simulink model "GUAM"  (R2023b)
settings: Solver=FixedStepAuto  StartTime=0.0  StopTime=SimIn.stopTime  FixedStep=Ts  RelTol=1e-3  AbsTol=1e-4  EnableMultiTasking=on
PostLoadFcn:
  | warning('off','sm:sli:setup:compile:LocalSolverNotSupported')
StartFcn:
  | tic
StopFcn:
  | Elapsed_Sim_Time = toc;
model workspace: external: MATLAB File aileronAssembly_DataFile.m (data not in the file)
values from neighbouring files (symbols this model uses):
  Ts = 0.05    [RUNME.m]
undefined symbols (not defined in the file or in its folder): AAC_Param, ang2Ext_coeff, Ki, Ki_scaling_elec, Kp, Leadscrew, motor_friction, R7_sctrl, sigbuilder_block, SimIn, SimPar, sm_aileron_actuator_lib, smiData, X, Y, Z
libraries: sm_lib x608, fl_lib x378, ee_lib x105, nesl_utility x96, simulink x10, eeGeneralControl x7, sh_lib x7, dspstat3 x6, sdl_lib x3, slpidlib x2, aerolibfltsims x2
(part 9 of 22)

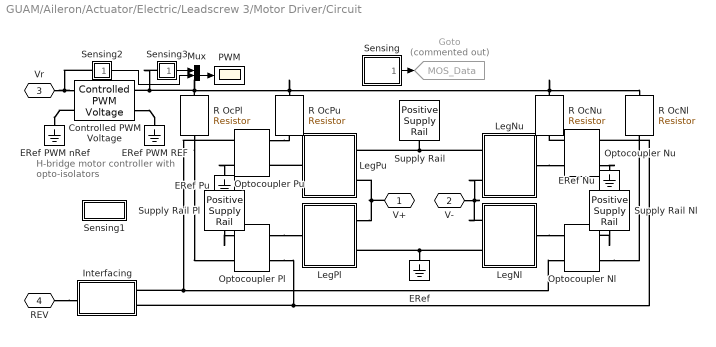
== system GUAM/Aileron/Actuator/Electric/Leadscrew 3/Motor Driver/Circuit ==
  note: H-bridge motor controller
      | with opto-isolators
  Controlled PWM Voltage : ee_lib/Integrated Circuits/Controlled PWM Voltage  F=10000 Hz  TD=0 s  pulse_width_offset=0 s  pulse_min=0 s  pwm_or_av=2  event_type=1  sample_time=1e-6 s  Vmin=0 V  Vmax=5 V  Vm=5 V  u_min=0  u_max=1
  ERef : fl_lib/Electrical/Electrical Elements/Electrical Reference
  ERef PWM REF : fl_lib/Electrical/Electrical Elements/Electrical Reference
  ERef PWM nRef : fl_lib/Electrical/Electrical Elements/Electrical Reference
  ERef Nu : fl_lib/Electrical/Electrical Elements/Electrical Reference
  ERef Pu : fl_lib/Electrical/Electrical Elements/Electrical Reference
  Goto : Goto  Commented=on  GotoTag=MOS_Data  TagVisibility=global
  Interfacing : Subsystem
  LegNl : Subsystem
      mask Display:
      | patch([96+30;0-30;0-30;96+30], [0+10;0+10;227-10;227-10], [1;1;1])
      | plot([96.6109160799533;96.4198282107139;95.8484048836359;94.9021492177306;93.5901741723367;91.9251147843401;89.9230064858609;87.6031306742773;84.9878290218281;82.1022883130956;78.9742978825019;75.6339819878271;72.1135096971394;68.4467850830839;64.6691207081296;60.8168975452888;56.927214609459;53.0375316736292;49.1853085107884;45.4076441358342;41.7409195217787;38.220447231091;34.8801313364162;31.7521409058224;28.86660019709;26.2512985446407;23.9314227330572;21.929314434578;20.2642550465813;18.9522800011875;18.0060243352822;17.4346010082041;17.2435131389648;17.4346010082041;18.0060243352822;18.9522800011875;20.2642550465814;21.9293144345781;23.9314227330573;26.2512985446408;28.8666001970901;31.7521409058226;34.8801313364163;38.2204472310911;41.7409195217788;45.4076441358342;49.1853085107884;53.0375316736292;56.927214609459;60.8168975452889;64.6691207081297;68.4467850830839;72.1135096971393;75.633981987827;78.9742978825018;82.1022883130955;84.9878290218281;87.6031306742773;89.9230064858608;91.9251147843399;93.5901741723367;94.9021492177305;95.8484048836358;96.4198282107139;96.6109160799533;96.6109160799533], [113.618216710165;109.728533774335;105.876310611494;102.09864623654;98.4319216224848;94.9114493317971;91.5711334371223;88.4431430065286;85.5576022977961;82.9423006453468;80.6224248337633;78.6203165352841;76.9552571472875;75.6432821018936;74.6970264359883;74.1256031089102;73.9345152396709;74.1256031089102;74.6970264359883;75.6432821018936;76.9552571472875;78.6203165352842;80.6224248337634;82.9423006453469;85.5576022977961;88.4431430065287;91.5711334371223;94.9114493317971;98.4319216224849;102.09864623654;105.876310611495;109.728533774335;113.618216710165;117.507899645995;121.360122808836;125.13778718379;128.804511797846;132.324984088533;135.665299983208;138.793290413802;141.678831122534;144.294132774983;146.614008586567;148.616116885046;150.281176273043;151.593151318437;152.539406984342;153.11083031142;153.301918180659;153.11083031142;152.539406984342;151.593151318437;150.281176273043;148.616116885046;146.614008586567;144.294132774983;141.678831122534;138.793290413802;135.665299983208;132.324984088533;128.804511797846;125.13778718379;121.360122808836;117.507899645995;113.618216710165;113.618216710165])
      | plot([33.9988537598401;34.5027737785131], [113.618216710165;113.618216710165])
      | plot([0.236212508752942;34.2508137691766], [113.618216710165;113.618216710165])
      | plot([34.2508137691766;34.2508137691766], [136.294617550448;90.9418158698827])
      | plot([45.5890141893178;45.5890141893178], [136.294617550448;90.9418158698827])
      | plot([45.5890141893178;68.2654150296003], [130.625517340377;130.625517340377])
      | plot([68.2654150296003;68.2654150296003], [130.625517340377;170.309218810871])
      | plot([68.2654150296003;93.776365974918], [170.309218810871;170.309218810871])
      | plot([45.5890141893178;68.2654150296003], [96.6109160799533;96.6109160799533])
      | plot([68.2654150296003;68.2654150296003], [96.6109160799533;56.927214609459])
      | plot([68.2654150296003;96.6109160799533], [56.927214609459;56.927214609459])
      | plot([45.5890141893178;68.2654150296003], [113.618216710165;113.618216710165])
      | plot([68.2654150296003;68.2654150296003], [130.618216710165;113.6109160799533])
      | plot([51.5963148195297;62.2581143993884;51.5963148195297], [124.956417130306;113.618216710165;102.280016290024])
  LegNu : Subsystem
      mask Display:
      | patch([96+30;0-30;0-30;96+30], [0+10;0+10;227-10;227-10], [1;1;1])
      | plot([96.6109160799533;96.4198282107139;95.8484048836359;94.9021492177306;93.5901741723367;91.9251147843401;89.9230064858609;87.6031306742773;84.9878290218281;82.1022883130956;78.9742978825019;75.6339819878271;72.1135096971394;68.4467850830839;64.6691207081296;60.8168975452888;56.927214609459;53.0375316736292;49.1853085107884;45.4076441358342;41.7409195217787;38.220447231091;34.8801313364162;31.7521409058224;28.86660019709;26.2512985446407;23.9314227330572;21.929314434578;20.2642550465813;18.9522800011875;18.0060243352822;17.4346010082041;17.2435131389648;17.4346010082041;18.0060243352822;18.9522800011875;20.2642550465814;21.9293144345781;23.9314227330573;26.2512985446408;28.8666001970901;31.7521409058226;34.8801313364163;38.2204472310911;41.7409195217788;45.4076441358342;49.1853085107884;53.0375316736292;56.927214609459;60.8168975452889;64.6691207081297;68.4467850830839;72.1135096971393;75.633981987827;78.9742978825018;82.1022883130955;84.9878290218281;87.6031306742773;89.9230064858608;91.9251147843399;93.5901741723367;94.9021492177305;95.8484048836358;96.4198282107139;96.6109160799533;96.6109160799533], [113.618216710165;109.728533774335;105.876310611494;102.09864623654;98.4319216224848;94.9114493317971;91.5711334371223;88.4431430065286;85.5576022977961;82.9423006453468;80.6224248337633;78.6203165352841;76.9552571472875;75.6432821018936;74.6970264359883;74.1256031089102;73.9345152396709;74.1256031089102;74.6970264359883;75.6432821018936;76.9552571472875;78.6203165352842;80.6224248337634;82.9423006453469;85.5576022977961;88.4431430065287;91.5711334371223;94.9114493317971;98.4319216224849;102.09864623654;105.876310611495;109.728533774335;113.618216710165;117.507899645995;121.360122808836;125.13778718379;128.804511797846;132.324984088533;135.665299983208;138.793290413802;141.678831122534;144.294132774983;146.614008586567;148.616116885046;150.281176273043;151.593151318437;152.539406984342;153.11083031142;153.301918180659;153.11083031142;152.539406984342;151.593151318437;150.281176273043;148.616116885046;146.614008586567;144.294132774983;141.678831122534;138.793290413802;135.665299983208;132.324984088533;128.804511797846;125.13778718379;121.360122808836;117.507899645995;113.618216710165;113.618216710165])
      | plot([33.9988537598401;34.5027737785131], [113.618216710165;113.618216710165])
      | plot([0.236212508752942;34.2508137691766], [113.618216710165;113.618216710165])
      | plot([34.2508137691766;34.2508137691766], [136.294617550448;90.9418158698827])
      | plot([45.5890141893178;45.5890141893178], [136.294617550448;90.9418158698827])
      | plot([45.5890141893178;68.2654150296003], [130.625517340377;130.625517340377])
      | plot([68.2654150296003;68.2654150296003], [130.625517340377;170.309218810871])
      | plot([68.2654150296003;93.776365974918], [170.309218810871;170.309218810871])
      | plot([45.5890141893178;68.2654150296003], [96.6109160799533;96.6109160799533])
      | plot([68.2654150296003;68.2654150296003], [96.6109160799533;56.927214609459])
      | plot([68.2654150296003;96.6109160799533], [56.927214609459;56.927214609459])
      | plot([45.5890141893178;68.2654150296003], [113.618216710165;113.618216710165])
      | plot([68.2654150296003;68.2654150296003], [130.618216710165;113.6109160799533])
      | plot([51.5963148195297;62.2581143993884;51.5963148195297], [124.956417130306;113.618216710165;102.280016290024])
  LegPl : Subsystem
      mask Display:
      | patch([96+30;0-30;0-30;96+30], [0+10;0+10;227-10;227-10], [1;1;1])
      | plot([96.6109160799533;96.4198282107139;95.8484048836359;94.9021492177306;93.5901741723367;91.9251147843401;89.9230064858609;87.6031306742773;84.9878290218281;82.1022883130956;78.9742978825019;75.6339819878271;72.1135096971394;68.4467850830839;64.6691207081296;60.8168975452888;56.927214609459;53.0375316736292;49.1853085107884;45.4076441358342;41.7409195217787;38.220447231091;34.8801313364162;31.7521409058224;28.86660019709;26.2512985446407;23.9314227330572;21.929314434578;20.2642550465813;18.9522800011875;18.0060243352822;17.4346010082041;17.2435131389648;17.4346010082041;18.0060243352822;18.9522800011875;20.2642550465814;21.9293144345781;23.9314227330573;26.2512985446408;28.8666001970901;31.7521409058226;34.8801313364163;38.2204472310911;41.7409195217788;45.4076441358342;49.1853085107884;53.0375316736292;56.927214609459;60.8168975452889;64.6691207081297;68.4467850830839;72.1135096971393;75.633981987827;78.9742978825018;82.1022883130955;84.9878290218281;87.6031306742773;89.9230064858608;91.9251147843399;93.5901741723367;94.9021492177305;95.8484048836358;96.4198282107139;96.6109160799533;96.6109160799533], [113.618216710165;109.728533774335;105.876310611494;102.09864623654;98.4319216224848;94.9114493317971;91.5711334371223;88.4431430065286;85.5576022977961;82.9423006453468;80.6224248337633;78.6203165352841;76.9552571472875;75.6432821018936;74.6970264359883;74.1256031089102;73.9345152396709;74.1256031089102;74.6970264359883;75.6432821018936;76.9552571472875;78.6203165352842;80.6224248337634;82.9423006453469;85.5576022977961;88.4431430065287;91.5711334371223;94.9114493317971;98.4319216224849;102.09864623654;105.876310611495;109.728533774335;113.618216710165;117.507899645995;121.360122808836;125.13778718379;128.804511797846;132.324984088533;135.665299983208;138.793290413802;141.678831122534;144.294132774983;146.614008586567;148.616116885046;150.281176273043;151.593151318437;152.539406984342;153.11083031142;153.301918180659;153.11083031142;152.539406984342;151.593151318437;150.281176273043;148.616116885046;146.614008586567;144.294132774983;141.678831122534;138.793290413802;135.665299983208;132.324984088533;128.804511797846;125.13778718379;121.360122808836;117.507899645995;113.618216710165;113.618216710165])
      | plot([33.9988537598401;34.5027737785131], [113.618216710165;113.618216710165])
      | plot([0.236212508752942;34.2508137691766], [113.618216710165;113.618216710165])
      | plot([34.2508137691766;34.2508137691766], [136.294617550448;90.9418158698827])
      | plot([45.5890141893178;45.5890141893178], [136.294617550448;90.9418158698827])
      | plot([45.5890141893178;68.2654150296003], [130.625517340377;130.625517340377])
      | plot([68.2654150296003;68.2654150296003], [130.625517340377;170.309218810871])
      | plot([68.2654150296003;93.776365974918], [170.309218810871;170.309218810871])
      | plot([45.5890141893178;68.2654150296003], [96.6109160799533;96.6109160799533])
      | plot([68.2654150296003;68.2654150296003], [96.6109160799533;56.927214609459])
      | plot([68.2654150296003;96.6109160799533], [56.927214609459;56.927214609459])
      | plot([45.5890141893178;68.2654150296003], [113.618216710165;113.618216710165])
      | plot([68.2654150296003;68.2654150296003], [130.618216710165;113.6109160799533])
      | plot([51.5963148195297;62.2581143993884;51.5963148195297], [124.956417130306;113.618216710165;102.280016290024])
  LegPu : Subsystem
      mask Display:
      | patch([96+30;0-30;0-30;96+30], [0+10;0+10;227-10;227-10], [1;1;1])
      | plot([96.6109160799533;96.4198282107139;95.8484048836359;94.9021492177306;93.5901741723367;91.9251147843401;89.9230064858609;87.6031306742773;84.9878290218281;82.1022883130956;78.9742978825019;75.6339819878271;72.1135096971394;68.4467850830839;64.6691207081296;60.8168975452888;56.927214609459;53.0375316736292;49.1853085107884;45.4076441358342;41.7409195217787;38.220447231091;34.8801313364162;31.7521409058224;28.86660019709;26.2512985446407;23.9314227330572;21.929314434578;20.2642550465813;18.9522800011875;18.0060243352822;17.4346010082041;17.2435131389648;17.4346010082041;18.0060243352822;18.9522800011875;20.2642550465814;21.9293144345781;23.9314227330573;26.2512985446408;28.8666001970901;31.7521409058226;34.8801313364163;38.2204472310911;41.7409195217788;45.4076441358342;49.1853085107884;53.0375316736292;56.927214609459;60.8168975452889;64.6691207081297;68.4467850830839;72.1135096971393;75.633981987827;78.9742978825018;82.1022883130955;84.9878290218281;87.6031306742773;89.9230064858608;91.9251147843399;93.5901741723367;94.9021492177305;95.8484048836358;96.4198282107139;96.6109160799533;96.6109160799533], [113.618216710165;109.728533774335;105.876310611494;102.09864623654;98.4319216224848;94.9114493317971;91.5711334371223;88.4431430065286;85.5576022977961;82.9423006453468;80.6224248337633;78.6203165352841;76.9552571472875;75.6432821018936;74.6970264359883;74.1256031089102;73.9345152396709;74.1256031089102;74.6970264359883;75.6432821018936;76.9552571472875;78.6203165352842;80.6224248337634;82.9423006453469;85.5576022977961;88.4431430065287;91.5711334371223;94.9114493317971;98.4319216224849;102.09864623654;105.876310611495;109.728533774335;113.618216710165;117.507899645995;121.360122808836;125.13778718379;128.804511797846;132.324984088533;135.665299983208;138.793290413802;141.678831122534;144.294132774983;146.614008586567;148.616116885046;150.281176273043;151.593151318437;152.539406984342;153.11083031142;153.301918180659;153.11083031142;152.539406984342;151.593151318437;150.281176273043;148.616116885046;146.614008586567;144.294132774983;141.678831122534;138.793290413802;135.665299983208;132.324984088533;128.804511797846;125.13778718379;121.360122808836;117.507899645995;113.618216710165;113.618216710165])
      | plot([33.9988537598401;34.5027737785131], [113.618216710165;113.618216710165])
      | plot([0.236212508752942;34.2508137691766], [113.618216710165;113.618216710165])
      | plot([34.2508137691766;34.2508137691766], [136.294617550448;90.9418158698827])
      | plot([45.5890141893178;45.5890141893178], [136.294617550448;90.9418158698827])
      | plot([45.5890141893178;68.2654150296003], [130.625517340377;130.625517340377])
      | plot([68.2654150296003;68.2654150296003], [130.625517340377;170.309218810871])
      | plot([68.2654150296003;93.776365974918], [170.309218810871;170.309218810871])
      | plot([45.5890141893178;68.2654150296003], [96.6109160799533;96.6109160799533])
      | plot([68.2654150296003;68.2654150296003], [96.6109160799533;56.927214609459])
      | plot([68.2654150296003;96.6109160799533], [56.927214609459;56.927214609459])
      | plot([45.5890141893178;68.2654150296003], [113.618216710165;113.618216710165])
      | plot([68.2654150296003;68.2654150296003], [130.618216710165;113.6109160799533])
      | plot([51.5963148195297;62.2581143993884;51.5963148195297], [124.956417130306;113.618216710165;102.280016290024])
  Mux : Mux  Inputs=2
  Optocoupler Nl : ee_lib/Semiconductors & Converters/Optocoupler  CTR=0.2  prmExp=1  I12="[  0.001 0.015 ] A"  V12="[  0.9 1.05 ] V"  IS=1e-10 A  ec=2  RS=0 Ohm  Tmeas=298.15 K  C_param=1  CJ=50 pF  CJ0=50 pF  VJ=1 V  Mgrad=0.5  Vvec="[  0.1 10 100 ] V"  Cvec="[  3.5 1 0.4 ] pF"  FC=0.5  T_param=1  IS_T2=1.8e-8 A  I1_T2=0.029 A  V1_T2=1.05 V  Tmeas2=125 degC  EG_param=1  EG=1.11 eV  XTI_param=1  XTI=3  Tdevice=25 degC  i_specify=off  i_priority=None  i=0 A  i_nominal_specify=off  i_nominal_unit=A  i_nominal_value=1  v_specify=off  v_priority=None  v=0 V  v_nominal_specify=off  v_nominal_unit=V  v_nominal_value=1  v_capacitor_specify=off  v_capacitor_priority=None  v_capacitor=0 V  v_capacitor_nominal_specify=off  v_capacitor_nominal_unit=V  v_capacitor_nominal_value=1  thermal_network_parameterization=ee.enum.thermalNetworkTopology.junctionCase  Rth=[0, 10] K/W  Rth_Cauer=[1, 3, 10] K/W  Rth_Foster=[4, 6] K/W  thermal_mass_parameterization=ee.enum.thermalNetwork.timeconstant  thermal_mass=[0, 1] J/K  thermal_mass_Cauer=[.1, .3, 1] J/K  thermal_mass_Foster=[1.5, 3] J/K  thermal_time_constant=[0, 10] s  thermal_time_constant_Cauer=[1, 3, 10] s  thermal_time_constant_Foster=[6, 18] s  thermal_mass_initial_temperatures=[25, 25] degC  thermal_mass_initial_temperatures_Cauer=[25, 25, 25] degC  Tvec_initial_Foster=[25, 25, 25, 25] degC  i_capacitor_specify=off  i_capacitor_priority=High  i_capacitor=0 A  i_capacitor_nominal_specify=off  i_capacitor_nominal_unit=A  i_capacitor_nominal_value=1
      settings: InternalSimscapePortConfiguration="{\"Bottom\":[],\"Left\":[{\"id\":\"p\",\"label\":\"\",\"type\":\"foundation.electrical.electrical\"},{\"id\":\"C\",\"label\":\"\",\"type\":\"foundation.electrical.electrical\"}],\"Right\":[{\"id\":\"n\",\"label\":\"\",\"type\":\"foundation.electrical.electrical\"},{\"id\":\"E\",\"label\":\"\",\"type\":\"foundation.electrical.electrical\"}],\"Top\":[]}"
  Optocoupler Nu : ee_lib/Semiconductors & Converters/Optocoupler  CTR=0.2  prmExp=1  I12="[  0.001 0.015 ] A"  V12="[  0.9 1.05 ] V"  IS=1e-10 A  ec=2  RS=0 Ohm  Tmeas=298.15 K  C_param=1  CJ=50 pF  CJ0=50 pF  VJ=1 V  Mgrad=0.5  Vvec="[  0.1 10 100 ] V"  Cvec="[  3.5 1 0.4 ] pF"  FC=0.5  T_param=1  IS_T2=1.8e-8 A  I1_T2=0.029 A  V1_T2=1.05 V  Tmeas2=125 degC  EG_param=1  EG=1.11 eV  XTI_param=1  XTI=3  Tdevice=25 degC  i_specify=off  i_priority=None  i=0 A  i_nominal_specify=off  i_nominal_unit=A  i_nominal_value=1  v_specify=off  v_priority=None  v=0 V  v_nominal_specify=off  v_nominal_unit=V  v_nominal_value=1  v_capacitor_specify=off  v_capacitor_priority=None  v_capacitor=0 V  v_capacitor_nominal_specify=off  v_capacitor_nominal_unit=V  v_capacitor_nominal_value=1  thermal_network_parameterization=ee.enum.thermalNetworkTopology.junctionCase  Rth=[0, 10] K/W  Rth_Cauer=[1, 3, 10] K/W  Rth_Foster=[4, 6] K/W  thermal_mass_parameterization=ee.enum.thermalNetwork.timeconstant  thermal_mass=[0, 1] J/K  thermal_mass_Cauer=[.1, .3, 1] J/K  thermal_mass_Foster=[1.5, 3] J/K  thermal_time_constant=[0, 10] s  thermal_time_constant_Cauer=[1, 3, 10] s  thermal_time_constant_Foster=[6, 18] s  thermal_mass_initial_temperatures=[25, 25] degC  thermal_mass_initial_temperatures_Cauer=[25, 25, 25] degC  Tvec_initial_Foster=[25, 25, 25, 25] degC  i_capacitor_specify=off  i_capacitor_priority=High  i_capacitor=0 A  i_capacitor_nominal_specify=off  i_capacitor_nominal_unit=A  i_capacitor_nominal_value=1
      settings: InternalSimscapePortConfiguration="{\"Bottom\":[],\"Left\":[{\"id\":\"p\",\"label\":\"\",\"type\":\"foundation.electrical.electrical\"},{\"id\":\"C\",\"label\":\"\",\"type\":\"foundation.electrical.electrical\"}],\"Right\":[{\"id\":\"n\",\"label\":\"\",\"type\":\"foundation.electrical.electrical\"},{\"id\":\"E\",\"label\":\"\",\"type\":\"foundation.electrical.electrical\"}],\"Top\":[]}"
  Optocoupler Pl : ee_lib/Semiconductors & Converters/Optocoupler  CTR=0.2  prmExp=1  I12="[  0.001 0.015 ] A"  V12="[  0.9 1.05 ] V"  IS=1e-10 A  ec=2  RS=0 Ohm  Tmeas=298.15 K  C_param=1  CJ=50 pF  CJ0=50 pF  VJ=1 V  Mgrad=0.5  Vvec="[  0.1 10 100 ] V"  Cvec="[  3.5 1 0.4 ] pF"  FC=0.5  T_param=1  IS_T2=1.8e-8 A  I1_T2=0.029 A  V1_T2=1.05 V  Tmeas2=125 degC  EG_param=1  EG=1.11 eV  XTI_param=1  XTI=3  Tdevice=25 degC  i_specify=off  i_priority=None  i=0 A  i_nominal_specify=off  i_nominal_unit=A  i_nominal_value=1  v_specify=off  v_priority=None  v=0 V  v_nominal_specify=off  v_nominal_unit=V  v_nominal_value=1  v_capacitor_specify=off  v_capacitor_priority=None  v_capacitor=0 V  v_capacitor_nominal_specify=off  v_capacitor_nominal_unit=V  v_capacitor_nominal_value=1  thermal_network_parameterization=ee.enum.thermalNetworkTopology.junctionCase  Rth=[0, 10] K/W  Rth_Cauer=[1, 3, 10] K/W  Rth_Foster=[4, 6] K/W  thermal_mass_parameterization=ee.enum.thermalNetwork.timeconstant  thermal_mass=[0, 1] J/K  thermal_mass_Cauer=[.1, .3, 1] J/K  thermal_mass_Foster=[1.5, 3] J/K  thermal_time_constant=[0, 10] s  thermal_time_constant_Cauer=[1, 3, 10] s  thermal_time_constant_Foster=[6, 18] s  thermal_mass_initial_temperatures=[25, 25] degC  thermal_mass_initial_temperatures_Cauer=[25, 25, 25] degC  Tvec_initial_Foster=[25, 25, 25, 25] degC  i_capacitor_specify=off  i_capacitor_priority=High  i_capacitor=0 A  i_capacitor_nominal_specify=off  i_capacitor_nominal_unit=A  i_capacitor_nominal_value=1
      settings: InternalSimscapePortConfiguration="{\"Bottom\":[],\"Left\":[{\"id\":\"p\",\"label\":\"\",\"type\":\"foundation.electrical.electrical\"},{\"id\":\"C\",\"label\":\"\",\"type\":\"foundation.electrical.electrical\"}],\"Right\":[{\"id\":\"n\",\"label\":\"\",\"type\":\"foundation.electrical.electrical\"},{\"id\":\"E\",\"label\":\"\",\"type\":\"foundation.electrical.electrical\"}],\"Top\":[]}"
  Optocoupler Pu : ee_lib/Semiconductors & Converters/Optocoupler  CTR=0.2  prmExp=1  I12="[  0.001 0.015 ] A"  V12="[  0.9 1.05 ] V"  IS=1e-10 A  ec=2  RS=0 Ohm  Tmeas=298.15 K  C_param=1  CJ=50 pF  CJ0=50 pF  VJ=1 V  Mgrad=0.5  Vvec="[  0.1 10 100 ] V"  Cvec="[  3.5 1 0.4 ] pF"  FC=0.5  T_param=1  IS_T2=1.8e-8 A  I1_T2=0.029 A  V1_T2=1.05 V  Tmeas2=125 degC  EG_param=1  EG=1.11 eV  XTI_param=1  XTI=3  Tdevice=25 degC  i_specify=off  i_priority=None  i=0 A  i_nominal_specify=off  i_nominal_unit=A  i_nominal_value=1  v_specify=off  v_priority=None  v=0 V  v_nominal_specify=off  v_nominal_unit=V  v_nominal_value=1  v_capacitor_specify=off  v_capacitor_priority=None  v_capacitor=0 V  v_capacitor_nominal_specify=off  v_capacitor_nominal_unit=V  v_capacitor_nominal_value=1  thermal_network_parameterization=ee.enum.thermalNetworkTopology.junctionCase  Rth=[0, 10] K/W  Rth_Cauer=[1, 3, 10] K/W  Rth_Foster=[4, 6] K/W  thermal_mass_parameterization=ee.enum.thermalNetwork.timeconstant  thermal_mass=[0, 1] J/K  thermal_mass_Cauer=[.1, .3, 1] J/K  thermal_mass_Foster=[1.5, 3] J/K  thermal_time_constant=[0, 10] s  thermal_time_constant_Cauer=[1, 3, 10] s  thermal_time_constant_Foster=[6, 18] s  thermal_mass_initial_temperatures=[25, 25] degC  thermal_mass_initial_temperatures_Cauer=[25, 25, 25] degC  Tvec_initial_Foster=[25, 25, 25, 25] degC  i_capacitor_specify=off  i_capacitor_priority=High  i_capacitor=0 A  i_capacitor_nominal_specify=off  i_capacitor_nominal_unit=A  i_capacitor_nominal_value=1
      settings: InternalSimscapePortConfiguration="{\"Bottom\":[],\"Left\":[{\"id\":\"p\",\"label\":\"\",\"type\":\"foundation.electrical.electrical\"},{\"id\":\"C\",\"label\":\"\",\"type\":\"foundation.electrical.electrical\"}],\"Right\":[{\"id\":\"n\",\"label\":\"\",\"type\":\"foundation.electrical.electrical\"},{\"id\":\"E\",\"label\":\"\",\"type\":\"foundation.electrical.electrical\"}],\"Top\":[]}"
  PWM : Scope
  R OcNl : fl_lib/Electrical/Electrical Elements/Resistor  R=470 Ohm  i_specify=off  i_priority=High  i=0 A  i_nominal_specify=off  i_nominal_unit=A  i_nominal_value=1  v_specify=off  v_priority=High  v=0 V  v_nominal_specify=off  v_nominal_unit=V  v_nominal_value=1
  R OcNu : fl_lib/Electrical/Electrical Elements/Resistor  R=470 Ohm  i_specify=off  i_priority=High  i=0 A  i_nominal_specify=off  i_nominal_unit=A  i_nominal_value=1  v_specify=off  v_priority=High  v=0 V  v_nominal_specify=off  v_nominal_unit=V  v_nominal_value=1
  R OcPl : fl_lib/Electrical/Electrical Elements/Resistor  R=470 Ohm  i_specify=off  i_priority=High  i=0 A  i_nominal_specify=off  i_nominal_unit=A  i_nominal_value=1  v_specify=off  v_priority=High  v=0 V  v_nominal_specify=off  v_nominal_unit=V  v_nominal_value=1
  R OcPu : fl_lib/Electrical/Electrical Elements/Resistor  R=470 Ohm  i_specify=off  i_priority=High  i=0 A  i_nominal_specify=off  i_nominal_unit=A  i_nominal_value=1  v_specify=off  v_priority=High  v=0 V  v_nominal_specify=off  v_nominal_unit=V  v_nominal_value=1
  Sensing : Subsystem
  Sensing1 : Subsystem
  Sensing2 : Subsystem
      mask Display: disp('V')
  Sensing3 : Subsystem
      mask Display: disp('V')
  Supply Rail : ee_lib/Sources/Positive Supply Rail  v0=24 V
      settings: InternalSimscapePortConfiguration="{\"Bottom\":[],\"Left\":[],\"Right\":[{\"id\":\"p\",\"label\":\"\",\"type\":\"foundation.electrical.electrical\"}],\"Top\":[]}"
  Supply Rail Nl : ee_lib/Sources/Positive Supply Rail  v0=24 V
      settings: InternalSimscapePortConfiguration="{\"Bottom\":[],\"Left\":[],\"Right\":[{\"id\":\"p\",\"label\":\"\",\"type\":\"foundation.electrical.electrical\"}],\"Top\":[]}"
  Supply Rail Pl : ee_lib/Sources/Positive Supply Rail  v0=24 V
      settings: InternalSimscapePortConfiguration="{\"Bottom\":[],\"Left\":[],\"Right\":[{\"id\":\"p\",\"label\":\"\",\"type\":\"foundation.electrical.electrical\"}],\"Top\":[]}"
  V+ : PMIOPort  Side=Right
  V- : PMIOPort  Port=2  Side=Right
  Vr : PMIOPort  Port=3  Side=Left
  REV : PMIOPort  Port=4  Side=Left
  wires:
  Sensing3/1(Out1) -> Mux/1
  Sensing2/1(Out1) -> Mux/2
  Mux/1 -> PWM/1
  Sensing/1(Data) -> Goto/1
  connections:
  LegPu/RConn2 -- V+/RConn1 -- LegPl/RConn1
  R OcPu/LConn1 -- R OcNl/RConn1 -- R OcNu/RConn1 -- Controlled PWM Voltage/RConn1 -- Sensing3/LConn1 -- R OcPl/RConn1
  LegPu/RConn1 -- Supply Rail/RConn1 -- LegNu/RConn1
  Optocoupler Pu/RConn1 -- Interfacing/RConn1 -- Optocoupler Nl/RConn1
  Optocoupler Pl/RConn1 -- Interfacing/RConn2 -- Optocoupler Nu/RConn1
  LegPl/RConn2 -- ERef/LConn1 -- LegNl/RConn2
  LegNu/RConn2 -- V-/RConn1 -- LegNl/RConn1
  LegPu/LConn1 -- Optocoupler Pu/LConn2
  Controlled PWM Voltage/RConn2 -- ERef PWM REF/LConn1
  Optocoupler Nu/LConn1 -- R OcNu/LConn1
  Supply Rail Pl/RConn1 -- Optocoupler Pl/LConn2
  LegNl/LConn1 -- Optocoupler Nl/RConn2
  Optocoupler Pu/RConn2 -- ERef Pu/LConn1
  Controlled PWM Voltage/LConn1 -- Sensing2/LConn1 -- Vr/RConn1
  Supply Rail Nl/RConn1 -- Optocoupler Nl/LConn2
  REV/RConn1 -- Interfacing/LConn1
  R OcPl/LConn1 -- Optocoupler Pl/LConn1
  Optocoupler Pl/RConn2 -- LegPl/LConn1
  LegNu/LConn1 -- Optocoupler Nu/LConn2
  Optocoupler Pu/LConn1 -- R OcPu/RConn1
  Controlled PWM Voltage/LConn2 -- ERef PWM nRef/LConn1
  Optocoupler Nu/RConn2 -- ERef Nu/LConn1
  Optocoupler Nl/LConn1 -- R OcNl/LConn1

== system GUAM/Aileron/Mechanical/Aileron_Att_1/MountC_Att_1/Bracket C/AilBrk_C_1_RIGID ==
  ReferenceFrame : sm_lib/Frames and Transforms/Reference Frame
  Solid : sm_lib/Body Elements/File Solid  ExtGeomFileName=AilBrk_C.step  UnitType=FromFile  ExtGeomFileUnits=m  StepReaderType=HEX  ExportConvexHullGeometry=off  InertiaType=Custom  Mass=smiData.Solid(15).mass  MassUnits=kg  CenterOfMass=smiData.Solid(15).CoM  CenterOfMassUnits=m  MomentsOfInertia=smiData.Solid(15).MoI  MomentsOfInertiaUnits=kg*m^2  ProductsOfInertia=smiData.Solid(15).PoI  ProductsOfInertiaUnits=kg*m^2  BasedOnType=Density  Density=1000  DensityUnits=kg/m^3  DoExposeReferenceFrame=on  SerializedFrames=<Frames/>  GraphicType=FromGeometry  MarkerShape=Sphere  MarkerSize=10  GraphicVisPropType=SimpleVisualProperties  GraphicDiffuseColor=smiData.Solid(15).color  GraphicSpecularColor=[0.5 0.5 0.5 1.0]  GraphicAmbientColor=[0.15 0.15 0.15 1.0]  GraphicEmissiveColor=[0.0 0.0 0.0 1.0]  GraphicShininess=75  GraphicOpacity=smiData.Solid(15).opacity
  Transform : sm_lib/Frames and Transforms/Rigid Transform  TranslationMethod=Cartesian  TranslationStandardOffset=0  TranslationStandardOffsetUnits=m  TranslationStandardAxis=+Z  TranslationCartesianOffset=smiData.RigidTransform(98).translation  TranslationCartesianOffsetUnits=m  TranslationROffset=0  TranslationROffsetUnits=m  TranslationZOffset=0  TranslationZOffsetUnits=m  TranslationThetaOffset=0  TranslationThetaOffsetUnits=deg  RotationMethod=ArbitraryAxis  RotationAngleUnits=rad  RotationStandardAxis=+Z  RotationAngle=smiData.RigidTransform(98).angle  RotationArbitraryAxis=smiData.RigidTransform(98).axis  FollAlignAxisA=+X  BaseAlignAxisA=+Y  FollAlignAxisB=+Y  BaseAlignAxisB=+Z  RotationSequenceAxes=FollowerAxes  RotationSequence=XYX  RotationSequenceAngles=[0 0 0]  RotationSequenceAnglesUnits=deg  RotationMatrix=[1 0 0; 0 1 0; 0 0 1]  Quaternion=[1 0 0 0]
  Transform Manual4Vis : sm_lib/Frames and Transforms/Rigid Transform  TranslationMethod=Cartesian  TranslationStandardOffset=0  TranslationStandardOffsetUnits=m  TranslationStandardAxis=+Z  TranslationCartesianOffset=[-1 1 0]*AAC_Param.AilBrk.LRManual4Vis  TranslationCartesianOffsetUnits=m  TranslationROffset=0  TranslationROffsetUnits=m  TranslationZOffset=0  TranslationZOffsetUnits=m  TranslationThetaOffset=0  TranslationThetaOffsetUnits=deg  RotationMethod=None  RotationAngleUnits=deg  RotationStandardAxis=+Z  RotationAngle=0.0  RotationArbitraryAxis=[0 0 1]  FollAlignAxisA=+X  BaseAlignAxisA=+Y  FollAlignAxisB=+Y  BaseAlignAxisB=+Z  RotationSequenceAxes=FollowerAxes  RotationSequence=XYX  RotationSequenceAngles=[0 0 0]  RotationSequenceAnglesUnits=deg  RotationMatrix=[1 0 0; 0 1 0; 0 0 1]  Quaternion=[1 0 0 0]
  Transform1 : sm_lib/Frames and Transforms/Rigid Transform  TranslationMethod=Cartesian  TranslationStandardOffset=0  TranslationStandardOffsetUnits=m  TranslationStandardAxis=+Z  TranslationCartesianOffset=smiData.RigidTransform(172).translation  TranslationCartesianOffsetUnits=m  TranslationROffset=0  TranslationROffsetUnits=m  TranslationZOffset=0  TranslationZOffsetUnits=m  TranslationThetaOffset=0  TranslationThetaOffsetUnits=deg  RotationMethod=ArbitraryAxis  RotationAngleUnits=rad  RotationStandardAxis=+Z  RotationAngle=smiData.RigidTransform(172).angle  RotationArbitraryAxis=smiData.RigidTransform(172).axis  FollAlignAxisA=+X  BaseAlignAxisA=+Y  FollAlignAxisB=+Y  BaseAlignAxisB=+Z  RotationSequenceAxes=FollowerAxes  RotationSequence=XYX  RotationSequenceAngles=[0 0 0]  RotationSequenceAnglesUnits=deg  RotationMatrix=[1 0 0; 0 1 0; 0 0 1]  Quaternion=[1 0 0 0]
  Transform2 : sm_lib/Frames and Transforms/Rigid Transform  TranslationMethod=Cartesian  TranslationStandardOffset=0  TranslationStandardOffsetUnits=m  TranslationStandardAxis=+Z  TranslationCartesianOffset=smiData.RigidTransform(200).translation  TranslationCartesianOffsetUnits=m  TranslationROffset=0  TranslationROffsetUnits=m  TranslationZOffset=0  TranslationZOffsetUnits=m  TranslationThetaOffset=0  TranslationThetaOffsetUnits=deg  RotationMethod=ArbitraryAxis  RotationAngleUnits=rad  RotationStandardAxis=+Z  RotationAngle=smiData.RigidTransform(200).angle  RotationArbitraryAxis=smiData.RigidTransform(200).axis  FollAlignAxisA=+X  BaseAlignAxisA=+Y  FollAlignAxisB=+Y  BaseAlignAxisB=+Z  RotationSequenceAxes=FollowerAxes  RotationSequence=XYX  RotationSequenceAngles=[0 0 0]  RotationSequenceAnglesUnits=deg  RotationMatrix=[1 0 0; 0 1 0; 0 0 1]  Quaternion=[1 0 0 0]
  G : PMIOPort  Side=Left
  F : PMIOPort  Port=2  Side=Right
  F1 : PMIOPort  Port=3  Side=Left
  connections:
  Transform Manual4Vis/RConn1 -- Solid/RConn1
  Transform/LConn1 -- G/RConn1
  Transform1/RConn1 -- F/RConn1
  Transform2/RConn1 -- F1/RConn1
  ReferenceFrame/RConn1 -- Transform1/LConn1 -- Transform2/LConn1 -- Transform Manual4Vis/LConn1 -- Transform/RConn1

== system GUAM/Aileron/Mechanical/Aileron_Att_1/MountC_Att_1/Bracket C/Bolt CBrk ==
  Hex_Flange_Screw_M6_1_RIGID : Subsystem
  Hex_Flange_Screw_M6_2_RIGID : Subsystem
  Hex_Flange_Screw_M6_3_RIGID : Subsystem
  Hex_Flange_Screw_M6_4_RIGID : Subsystem
  Hex_Flange_Screw_M6_5_RIGID : Subsystem
  Hex_Flange_Screw_M6_6_RIGID : Subsystem
  G : PMIOPort  Side=Left
  connections:
  Hex_Flange_Screw_M6_6_RIGID/LConn1 -- Hex_Flange_Screw_M6_5_RIGID/LConn1 -- G/RConn1 -- Hex_Flange_Screw_M6_1_RIGID/LConn1 -- Hex_Flange_Screw_M6_2_RIGID/LConn1 -- Hex_Flange_Screw_M6_3_RIGID/LConn1 -- Hex_Flange_Screw_M6_4_RIGID/LConn1

== system GUAM/Aileron/Mechanical/Aileron_Att_1/MountC_Att_1/Bracket C/Screws CBrk ==
  Hex_Bolt_M10_3_RIGID : Subsystem
  Hex_Flange_Nut_M10_1_RIGID : Subsystem
  Washer_3_RIGID : Subsystem
  Washer_4_RIGID : Subsystem
  G : PMIOPort  Side=Left
  connections:
  Hex_Bolt_M10_3_RIGID/LConn1 -- G/RConn1 -- Washer_4_RIGID/LConn1 -- Washer_3_RIGID/LConn1 -- Hex_Flange_Nut_M10_1_RIGID/LConn1

== system GUAM/Aileron/Mechanical/Aileron_Att_1/MountC_Att_1/Bracket L/AilBrk_L_1_RIGID ==
  ReferenceFrame : sm_lib/Frames and Transforms/Reference Frame
  Solid : sm_lib/Body Elements/File Solid  ExtGeomFileName=AilBrk_L.step  UnitType=FromFile  ExtGeomFileUnits=m  StepReaderType=HEX  ExportConvexHullGeometry=off  InertiaType=Custom  Mass=smiData.Solid(13).mass  MassUnits=kg  CenterOfMass=smiData.Solid(13).CoM  CenterOfMassUnits=m  MomentsOfInertia=smiData.Solid(13).MoI  MomentsOfInertiaUnits=kg*m^2  ProductsOfInertia=smiData.Solid(13).PoI  ProductsOfInertiaUnits=kg*m^2  BasedOnType=Density  Density=1000  DensityUnits=kg/m^3  DoExposeReferenceFrame=on  SerializedFrames=<Frames/>  GraphicType=FromGeometry  MarkerShape=Sphere  MarkerSize=10  GraphicVisPropType=SimpleVisualProperties  GraphicDiffuseColor=smiData.Solid(13).color  GraphicSpecularColor=[0.5 0.5 0.5 1.0]  GraphicAmbientColor=[0.15 0.15 0.15 1.0]  GraphicEmissiveColor=[0.0 0.0 0.0 1.0]  GraphicShininess=75  GraphicOpacity=smiData.Solid(13).opacity
  Transform : sm_lib/Frames and Transforms/Rigid Transform  TranslationMethod=Cartesian  TranslationStandardOffset=0  TranslationStandardOffsetUnits=m  TranslationStandardAxis=+Z  TranslationCartesianOffset=smiData.RigidTransform(103).translation  TranslationCartesianOffsetUnits=m  TranslationROffset=0  TranslationROffsetUnits=m  TranslationZOffset=0  TranslationZOffsetUnits=m  TranslationThetaOffset=0  TranslationThetaOffsetUnits=deg  RotationMethod=ArbitraryAxis  RotationAngleUnits=rad  RotationStandardAxis=+Z  RotationAngle=smiData.RigidTransform(103).angle  RotationArbitraryAxis=smiData.RigidTransform(103).axis  FollAlignAxisA=+X  BaseAlignAxisA=+Y  FollAlignAxisB=+Y  BaseAlignAxisB=+Z  RotationSequenceAxes=FollowerAxes  RotationSequence=XYX  RotationSequenceAngles=[0 0 0]  RotationSequenceAnglesUnits=deg  RotationMatrix=[1 0 0; 0 1 0; 0 0 1]  Quaternion=[1 0 0 0]
  Transform Manual4Vis : sm_lib/Frames and Transforms/Rigid Transform  TranslationMethod=StandardAxis  TranslationStandardOffset=AAC_Param.AilBrk.LRManual4Vis  TranslationStandardOffsetUnits=m  TranslationStandardAxis=+Y  TranslationCartesianOffset=[0 0 0]  TranslationCartesianOffsetUnits=m  TranslationROffset=0  TranslationROffsetUnits=m  TranslationZOffset=0  TranslationZOffsetUnits=m  TranslationThetaOffset=0  TranslationThetaOffsetUnits=deg  RotationMethod=None  RotationAngleUnits=deg  RotationStandardAxis=+Z  RotationAngle=0.0  RotationArbitraryAxis=[0 0 1]  FollAlignAxisA=+X  BaseAlignAxisA=+Y  FollAlignAxisB=+Y  BaseAlignAxisB=+Z  RotationSequenceAxes=FollowerAxes  RotationSequence=XYX  RotationSequenceAngles=[0 0 0]  RotationSequenceAnglesUnits=deg  RotationMatrix=[1 0 0; 0 1 0; 0 0 1]  Quaternion=[1 0 0 0]
  Transform1 : sm_lib/Frames and Transforms/Rigid Transform  TranslationMethod=Cartesian  TranslationStandardOffset=0  TranslationStandardOffsetUnits=m  TranslationStandardAxis=+Z  TranslationCartesianOffset=smiData.RigidTransform(174).translation  TranslationCartesianOffsetUnits=m  TranslationROffset=0  TranslationROffsetUnits=m  TranslationZOffset=0  TranslationZOffsetUnits=m  TranslationThetaOffset=0  TranslationThetaOffsetUnits=deg  RotationMethod=ArbitraryAxis  RotationAngleUnits=rad  RotationStandardAxis=+Z  RotationAngle=smiData.RigidTransform(174).angle  RotationArbitraryAxis=smiData.RigidTransform(174).axis  FollAlignAxisA=+X  BaseAlignAxisA=+Y  FollAlignAxisB=+Y  BaseAlignAxisB=+Z  RotationSequenceAxes=FollowerAxes  RotationSequence=XYX  RotationSequenceAngles=[0 0 0]  RotationSequenceAnglesUnits=deg  RotationMatrix=[1 0 0; 0 1 0; 0 0 1]  Quaternion=[1 0 0 0]
  G : PMIOPort  Side=Left
  F : PMIOPort  Port=2  Side=Right
  connections:
  Transform Manual4Vis/LConn1 -- ReferenceFrame/RConn1 -- Transform1/LConn1 -- Transform/RConn1
  Transform/LConn1 -- G/RConn1
  Transform1/RConn1 -- F/RConn1
  Transform Manual4Vis/RConn1 -- Solid/RConn1

== system GUAM/Aileron/Mechanical/Aileron_Att_1/MountC_Att_1/Bracket L/Bolt LBrk ==
  Hex_Bolt_M10_2_RIGID : Subsystem
  Washer_1_RIGID : Subsystem
  M : PMIOPort  Side=Left
  G : PMIOPort  Port=2  Side=Left
  connections:
  Washer_1_RIGID/LConn2 -- Hex_Bolt_M10_2_RIGID/LConn1 -- G/RConn1
  Washer_1_RIGID/LConn1 -- M/RConn1

== system GUAM/Aileron/Mechanical/Aileron_Att_1/MountC_Att_1/Bracket L/Screws LBrk ==
  Oval_Head_M4_12_RIGID : Subsystem
  Oval_Head_M4_1_RIGID : Subsystem
  Oval_Head_M4_4_RIGID : Subsystem
  Oval_Head_M4_5_RIGID : Subsystem
  Oval_Head_M4_6_RIGID : Subsystem
  Oval_Head_M4_8_RIGID : Subsystem
  G : PMIOPort  Side=Left
  connections:
  Oval_Head_M4_1_RIGID/LConn1 -- G/RConn1 -- Oval_Head_M4_8_RIGID/LConn1 -- Oval_Head_M4_6_RIGID/LConn1 -- Oval_Head_M4_5_RIGID/LConn1 -- Oval_Head_M4_4_RIGID/LConn1 -- Oval_Head_M4_12_RIGID/LConn1

== system GUAM/Aileron/Mechanical/Aileron_Att_1/MountC_Att_1/Bracket R/AilBrk_R_1_RIGID ==
  ReferenceFrame : sm_lib/Frames and Transforms/Reference Frame
  Solid : sm_lib/Body Elements/File Solid  ExtGeomFileName=AilBrk_R.step  UnitType=FromFile  ExtGeomFileUnits=m  StepReaderType=HEX  ExportConvexHullGeometry=off  InertiaType=Custom  Mass=smiData.Solid(16).mass  MassUnits=kg  CenterOfMass=smiData.Solid(16).CoM  CenterOfMassUnits=m  MomentsOfInertia=smiData.Solid(16).MoI  MomentsOfInertiaUnits=kg*m^2  ProductsOfInertia=smiData.Solid(16).PoI  ProductsOfInertiaUnits=kg*m^2  BasedOnType=Density  Density=1000  DensityUnits=kg/m^3  DoExposeReferenceFrame=on  SerializedFrames=<Frames/>  GraphicType=FromGeometry  MarkerShape=Sphere  MarkerSize=10  GraphicVisPropType=SimpleVisualProperties  GraphicDiffuseColor=smiData.Solid(16).color  GraphicSpecularColor=[0.5 0.5 0.5 1.0]  GraphicAmbientColor=[0.15 0.15 0.15 1.0]  GraphicEmissiveColor=[0.0 0.0 0.0 1.0]  GraphicShininess=75  GraphicOpacity=smiData.Solid(16).opacity
  Transform : sm_lib/Frames and Transforms/Rigid Transform  TranslationMethod=Cartesian  TranslationStandardOffset=0  TranslationStandardOffsetUnits=m  TranslationStandardAxis=+Z  TranslationCartesianOffset=smiData.RigidTransform(82).translation  TranslationCartesianOffsetUnits=m  TranslationROffset=0  TranslationROffsetUnits=m  TranslationZOffset=0  TranslationZOffsetUnits=m  TranslationThetaOffset=0  TranslationThetaOffsetUnits=deg  RotationMethod=ArbitraryAxis  RotationAngleUnits=rad  RotationStandardAxis=+Z  RotationAngle=smiData.RigidTransform(82).angle  RotationArbitraryAxis=smiData.RigidTransform(82).axis  FollAlignAxisA=+X  BaseAlignAxisA=+Y  FollAlignAxisB=+Y  BaseAlignAxisB=+Z  RotationSequenceAxes=FollowerAxes  RotationSequence=XYX  RotationSequenceAngles=[0 0 0]  RotationSequenceAnglesUnits=deg  RotationMatrix=[1 0 0; 0 1 0; 0 0 1]  Quaternion=[1 0 0 0]
  Transform Manual4Vis : sm_lib/Frames and Transforms/Rigid Transform  TranslationMethod=StandardAxis  TranslationStandardOffset=AAC_Param.AilBrk.LRManual4Vis  TranslationStandardOffsetUnits=m  TranslationStandardAxis=-Y  TranslationCartesianOffset=[0 0 0]  TranslationCartesianOffsetUnits=m  TranslationROffset=0  TranslationROffsetUnits=m  TranslationZOffset=0  TranslationZOffsetUnits=m  TranslationThetaOffset=0  TranslationThetaOffsetUnits=deg  RotationMethod=None  RotationAngleUnits=deg  RotationStandardAxis=+Z  RotationAngle=0.0  RotationArbitraryAxis=[0 0 1]  FollAlignAxisA=+X  BaseAlignAxisA=+Y  FollAlignAxisB=+Y  BaseAlignAxisB=+Z  RotationSequenceAxes=FollowerAxes  RotationSequence=XYX  RotationSequenceAngles=[0 0 0]  RotationSequenceAnglesUnits=deg  RotationMatrix=[1 0 0; 0 1 0; 0 0 1]  Quaternion=[1 0 0 0]
  Transform1 : sm_lib/Frames and Transforms/Rigid Transform  TranslationMethod=Cartesian  TranslationStandardOffset=0  TranslationStandardOffsetUnits=m  TranslationStandardAxis=+Z  TranslationCartesianOffset=smiData.RigidTransform(176).translation  TranslationCartesianOffsetUnits=m  TranslationROffset=0  TranslationROffsetUnits=m  TranslationZOffset=0  TranslationZOffsetUnits=m  TranslationThetaOffset=0  TranslationThetaOffsetUnits=deg  RotationMethod=ArbitraryAxis  RotationAngleUnits=rad  RotationStandardAxis=+Z  RotationAngle=smiData.RigidTransform(176).angle  RotationArbitraryAxis=smiData.RigidTransform(176).axis  FollAlignAxisA=+X  BaseAlignAxisA=+Y  FollAlignAxisB=+Y  BaseAlignAxisB=+Z  RotationSequenceAxes=FollowerAxes  RotationSequence=XYX  RotationSequenceAngles=[0 0 0]  RotationSequenceAnglesUnits=deg  RotationMatrix=[1 0 0; 0 1 0; 0 0 1]  Quaternion=[1 0 0 0]
  G : PMIOPort  Side=Left
  F : PMIOPort  Port=2  Side=Right
  connections:
  Transform Manual4Vis/LConn1 -- ReferenceFrame/RConn1 -- Transform1/LConn1 -- Transform/RConn1
  Transform/LConn1 -- G/RConn1
  Transform1/RConn1 -- F/RConn1
  Transform Manual4Vis/RConn1 -- Solid/RConn1

== system GUAM/Aileron/Mechanical/Aileron_Att_1/MountC_Att_1/Bracket R/Bolt RBrk ==
  Hex_Bolt_M10_1_RIGID : Subsystem
  Washer_2_RIGID : Subsystem
  G : PMIOPort  Side=Left
  connections:
  Hex_Bolt_M10_1_RIGID/LConn1 -- G/RConn1 -- Washer_2_RIGID/LConn1

== system GUAM/Aileron/Mechanical/Aileron_Att_1/MountC_Att_1/Bracket R/Screws RBrk ==
  Oval_Head_M4_10_RIGID : Subsystem
  Oval_Head_M4_11_RIGID : Subsystem
  Oval_Head_M4_2_RIGID : Subsystem
  Oval_Head_M4_3_RIGID : Subsystem
  Oval_Head_M4_7_RIGID : Subsystem
  Oval_Head_M4_9_RIGID : Subsystem
  G : PMIOPort  Side=Left
  connections:
  Oval_Head_M4_3_RIGID/LConn1 -- G/RConn1 -- Oval_Head_M4_10_RIGID/LConn1 -- Oval_Head_M4_11_RIGID/LConn1 -- Oval_Head_M4_2_RIGID/LConn1 -- Oval_Head_M4_9_RIGID/LConn1 -- Oval_Head_M4_7_RIGID/LConn1

== system GUAM/Aileron/Mechanical/Aileron_Att_1/MountL_Att_1/Bracket C/AilBrk_C_1_RIGID ==
  ReferenceFrame : sm_lib/Frames and Transforms/Reference Frame
  Solid : sm_lib/Body Elements/File Solid  ExtGeomFileName=AilBrk_C.step  UnitType=FromFile  ExtGeomFileUnits=m  StepReaderType=HEX  ExportConvexHullGeometry=off  InertiaType=Custom  Mass=smiData.Solid(15).mass  MassUnits=kg  CenterOfMass=smiData.Solid(15).CoM  CenterOfMassUnits=m  MomentsOfInertia=smiData.Solid(15).MoI  MomentsOfInertiaUnits=kg*m^2  ProductsOfInertia=smiData.Solid(15).PoI  ProductsOfInertiaUnits=kg*m^2  BasedOnType=Density  Density=1000  DensityUnits=kg/m^3  DoExposeReferenceFrame=on  SerializedFrames=<Frames/>  GraphicType=FromGeometry  MarkerShape=Sphere  MarkerSize=10  GraphicVisPropType=SimpleVisualProperties  GraphicDiffuseColor=smiData.Solid(15).color  GraphicSpecularColor=[0.5 0.5 0.5 1.0]  GraphicAmbientColor=[0.15 0.15 0.15 1.0]  GraphicEmissiveColor=[0.0 0.0 0.0 1.0]  GraphicShininess=75  GraphicOpacity=smiData.Solid(15).opacity
  Transform : sm_lib/Frames and Transforms/Rigid Transform  TranslationMethod=Cartesian  TranslationStandardOffset=0  TranslationStandardOffsetUnits=m  TranslationStandardAxis=+Z  TranslationCartesianOffset=smiData.RigidTransform(161).translation  TranslationCartesianOffsetUnits=m  TranslationROffset=0  TranslationROffsetUnits=m  TranslationZOffset=0  TranslationZOffsetUnits=m  TranslationThetaOffset=0  TranslationThetaOffsetUnits=deg  RotationMethod=ArbitraryAxis  RotationAngleUnits=rad  RotationStandardAxis=+Z  RotationAngle=smiData.RigidTransform(161).angle  RotationArbitraryAxis=smiData.RigidTransform(161).axis  FollAlignAxisA=+X  BaseAlignAxisA=+Y  FollAlignAxisB=+Y  BaseAlignAxisB=+Z  RotationSequenceAxes=FollowerAxes  RotationSequence=XYX  RotationSequenceAngles=[0 0 0]  RotationSequenceAnglesUnits=deg  RotationMatrix=[1 0 0; 0 1 0; 0 0 1]  Quaternion=[1 0 0 0]
  Transform Manual4Vis : sm_lib/Frames and Transforms/Rigid Transform  TranslationMethod=Cartesian  TranslationStandardOffset=0  TranslationStandardOffsetUnits=m  TranslationStandardAxis=+Z  TranslationCartesianOffset=[-1 1 0]*AAC_Param.AilBrk.LRManual4Vis  TranslationCartesianOffsetUnits=m  TranslationROffset=0  TranslationROffsetUnits=m  TranslationZOffset=0  TranslationZOffsetUnits=m  TranslationThetaOffset=0  TranslationThetaOffsetUnits=deg  RotationMethod=None  RotationAngleUnits=deg  RotationStandardAxis=+Z  RotationAngle=0.0  RotationArbitraryAxis=[0 0 1]  FollAlignAxisA=+X  BaseAlignAxisA=+Y  FollAlignAxisB=+Y  BaseAlignAxisB=+Z  RotationSequenceAxes=FollowerAxes  RotationSequence=XYX  RotationSequenceAngles=[0 0 0]  RotationSequenceAnglesUnits=deg  RotationMatrix=[1 0 0; 0 1 0; 0 0 1]  Quaternion=[1 0 0 0]
  Transform1 : sm_lib/Frames and Transforms/Rigid Transform  TranslationMethod=Cartesian  TranslationStandardOffset=0  TranslationStandardOffsetUnits=m  TranslationStandardAxis=+Z  TranslationCartesianOffset=smiData.RigidTransform(185).translation  TranslationCartesianOffsetUnits=m  TranslationROffset=0  TranslationROffsetUnits=m  TranslationZOffset=0  TranslationZOffsetUnits=m  TranslationThetaOffset=0  TranslationThetaOffsetUnits=deg  RotationMethod=ArbitraryAxis  RotationAngleUnits=rad  RotationStandardAxis=+Z  RotationAngle=smiData.RigidTransform(185).angle  RotationArbitraryAxis=smiData.RigidTransform(185).axis  FollAlignAxisA=+X  BaseAlignAxisA=+Y  FollAlignAxisB=+Y  BaseAlignAxisB=+Z  RotationSequenceAxes=FollowerAxes  RotationSequence=XYX  RotationSequenceAngles=[0 0 0]  RotationSequenceAnglesUnits=deg  RotationMatrix=[1 0 0; 0 1 0; 0 0 1]  Quaternion=[1 0 0 0]
  Transform2 : sm_lib/Frames and Transforms/Rigid Transform  TranslationMethod=Cartesian  TranslationStandardOffset=0  TranslationStandardOffsetUnits=m  TranslationStandardAxis=+Z  TranslationCartesianOffset=smiData.RigidTransform(202).translation  TranslationCartesianOffsetUnits=m  TranslationROffset=0  TranslationROffsetUnits=m  TranslationZOffset=0  TranslationZOffsetUnits=m  TranslationThetaOffset=0  TranslationThetaOffsetUnits=deg  RotationMethod=ArbitraryAxis  RotationAngleUnits=rad  RotationStandardAxis=+Z  RotationAngle=smiData.RigidTransform(202).angle  RotationArbitraryAxis=smiData.RigidTransform(202).axis  FollAlignAxisA=+X  BaseAlignAxisA=+Y  FollAlignAxisB=+Y  BaseAlignAxisB=+Z  RotationSequenceAxes=FollowerAxes  RotationSequence=XYX  RotationSequenceAngles=[0 0 0]  RotationSequenceAnglesUnits=deg  RotationMatrix=[1 0 0; 0 1 0; 0 0 1]  Quaternion=[1 0 0 0]
  G : PMIOPort  Side=Left
  F : PMIOPort  Port=2  Side=Right
  F1 : PMIOPort  Port=3  Side=Left
  connections:
  Transform Manual4Vis/LConn1 -- ReferenceFrame/RConn1 -- Transform1/LConn1 -- Transform2/LConn1 -- Transform/RConn1
  Transform/LConn1 -- G/RConn1
  Transform1/RConn1 -- F/RConn1
  Transform2/RConn1 -- F1/RConn1
  Transform Manual4Vis/RConn1 -- Solid/RConn1

== system GUAM/Aileron/Mechanical/Aileron_Att_1/MountL_Att_1/Bracket C/Bolt CBrk ==
  Hex_Bolt_M10_3_RIGID : Subsystem
  Hex_Flange_Nut_M10_1_RIGID : Subsystem
  Washer_1_RIGID : Subsystem
  Washer_4_RIGID : Subsystem
  G : PMIOPort  Side=Left
  connections:
  Hex_Flange_Nut_M10_1_RIGID/LConn1 -- G/RConn1 -- Hex_Bolt_M10_3_RIGID/LConn1 -- Washer_1_RIGID/LConn1 -- Washer_4_RIGID/LConn1

== system GUAM/Aileron/Mechanical/Aileron_Att_1/MountL_Att_1/Bracket C/Screws CBrk ==
  Hex_Flange_Screw_M6_1_RIGID : Subsystem
  Hex_Flange_Screw_M6_2_RIGID : Subsystem
  Hex_Flange_Screw_M6_3_RIGID : Subsystem
  Hex_Flange_Screw_M6_4_RIGID : Subsystem
  Hex_Flange_Screw_M6_5_RIGID : Subsystem
  Hex_Flange_Screw_M6_6_RIGID : Subsystem
  G : PMIOPort  Side=Left
  connections:
  Hex_Flange_Screw_M6_6_RIGID/LConn1 -- G/RConn1 -- Hex_Flange_Screw_M6_1_RIGID/LConn1 -- Hex_Flange_Screw_M6_2_RIGID/LConn1 -- Hex_Flange_Screw_M6_3_RIGID/LConn1 -- Hex_Flange_Screw_M6_4_RIGID/LConn1 -- Hex_Flange_Screw_M6_5_RIGID/LConn1
